simulink model "Test_model_671203"  (R2024a)
settings: Solver=VariableStepAuto  StartTime=0.0  StopTime=10  RelTol=1e-3
undefined symbols (not defined in the file or in its folder): X, Y, Z
libraries: sm_lib x63, nesl_utility x21
(part 3 of 3)

== matlab function Test_model_671203/MATLAB Function1 ==
  data: joint_angles input; x output; y output; z output
function [x, y, z] = FK_Simulink(joint_angles)
    % FK_Simulink: Calculates the position and orientation of the end effector for a 4-DOF manipulator

    % Lengths of the links
    d1 = 0.3;  % {0} -> {1}
    a1 = 0.2;  % {1} -> {2}
    L1 = 0.25; % Link 1
    L2 = 1;    % Link 2
    L3 = 1.5;  % Link 3
    L4 = 0.75; % Link 4 (End Effector)

    % Extract joint angles
    q1 = joint_angles(1); % Joint 1 (base rotation)
    q2 = joint_angles(2); % Joint 2 (shoulder rotation)
    q3 = joint_angles(3); % Joint 3 (elbow rotation)
    q4 = joint_angles(4); % Joint 4 (end effector orientation)

    x12 = pi/2;
    z23 = pi/2;

    % Transformation Matrices
    % Transform from base frame to end effector
    % Transformation for Joint 0 -> 1 (Rotation around the base)
    T01_T1 = [  1, 0, 0,  0;
                0, 1, 0,  0;
                0, 0, 1, d1;
                0, 0, 0,  1];

    T01_Rz = [  cos(q1), -sin(q1), 0, 0;
                sin(q1),  cos(q1), 0, 0;
                      0,        0, 1, 0;
                      0,        0, 0, 1];

    T01 = T01_T1 * T01_Rz;

    % Transformation for Joint 1 -> 2 (shoulder)
    T12_T1 = [  1, 0, 0, -a1;
                0, 1, 0,   0;
                0, 0, 1,  L1;
                0, 0, 0,   1];

    T12_Rx = [  1,        0,         0, 0;
                0, cos(x12), -sin(x12), 0;
                0, sin(x12),  cos(x12), 0;
                0,        0,         0, 1];

    T12_Rz = [  cos(q2), -sin(q2), 0, 0;
                sin(q2),  cos(q2), 0, 0;
                      0,        0, 1, 0;
                      0,        0, 0, 1];

    T12 = T12_T1 * T12_Rx * T12_Rz;

    % Transformation for Joint 2 -> 3 (elbow)
    T23_Rz1 = [  cos(z23), -sin(z23), 0, 0;
                 sin(z23),  cos(z23), 0, 0;
                        0,         0, 1, 0;
                        0,         0, 0, 1];

    T23_T1 = [  1, 0, 0, L2;
                0, 1, 0,  0;
                0, 0, 1,  0;
                0, 0, 0,  1];

    T23_Rz = [  cos(q3), -sin(q3), 0, 0;
                sin(q3),  cos(q3), 0, 0;
                      0,        0, 1, 0;
                      0,        0, 0, 1];

    T23 = T23_Rz1 * T23_T1 * T23_Rz;

    % Transformation for Joint 3 -> 4
    T34_T1 = [  1, 0, 0, L3;
                0, 1, 0,  0;
                0, 0, 1,  0;
                0, 0, 0,  1];

    T34_Rz = [  cos(q4), -sin(q4), 0, 0;
                sin(q4),  cos(q4), 0, 0;
                      0,        0, 1, 0;
                      0,        0, 0, 1];

    T34 = T34_T1 * T34_Rz;

    % Transformation for Joint 4 -> e

    T4e = [ 1, 0, 0, L4;
            0, 1, 0,  0;
            0, 0, 1,  0;
            0, 0, 0,  1];

    % Final transformation from the base to end effector
    T = T01 * T12 * T23 * T34 * T4e;

    % Extract position from the final transformation matrix
    x = T(1, 4); % x-position of the end effector
    y = T(2, 4); % y-position of the end effector
    z = T(3, 4); % z-position of the end effector

  
end

% Tranformation matrix
% ([  [-sin(q2 + q3 + q4)*cos(q1), -cos(q1)*cos(q2 + q3 + q4),  sin(q1), -L2*sin(q2)*cos(q1) - L3*sin(q2 + q3)*cos(q1) - L4*sin(q2 + q3 + q4)*cos(q1) - a1*cos(q1)], ...
%     [-sin(q1)*sin(q2 + q3 + q4), -sin(q1)*cos(q2 + q3 + q4), -cos(q1), -L2*sin(q1)*sin(q2) - L3*sin(q1)*sin(q2 + q3) - L4*sin(q1)*sin(q2 + q3 + q4) - a1*sin(q1)], ...
%     [         cos(q2 + q3 + q4),         -sin(q2 + q3 + q4),        0,                     L1 + L2*cos(q2) + L3*(1.0*cos(q2 + q3)) + L4*(cos(q2 + q3 + q4)) + d1], ...
%     [                         0,                          0,        0,                                                                                         1]  ])


function q = solveMatrix(x, y, z, phi)
    % Define matrices A, B, C, D, E (as 4x4 symbolic matrices)
    syms x y z phi real;
    
     % Lengths of the links
    d1 = 0.3;  % {0} -> {1}
    a1 = 0.2;  % {1} -> {2}
    L1 = 0.25; % Link 1
    L2 = 1;    % Link 2
    L3 = 1.5;  % Link 3
    L4 = 0.75; % Link 4 (End Effector)

    % Extract joint angles
    q1 = joint_angles(1); % Joint 1 (base rotation)
    q2 = joint_angles(2); % Joint 2 (shoulder rotation)
    q3 = joint_angles(3); % Joint 3 (elbow rotation)
    q4 = joint_angles(4); % Joint 4 (end effector orientation)

    x12 = pi/2;
    z23 = pi/2;

    % Transformation Matrices
    % Transform from base frame to end effector
    % Transformation for Joint 0 -> 1 (Rotation around the base)
    T01_T1 = [  1, 0, 0,  0;
                0, 1, 0,  0;
                0, 0, 1, d1;
                0, 0, 0,  1];

    T01_Rz = [  cos(q1), -sin(q1), 0, 0;
                sin(q1),  cos(q1), 0, 0;
                      0,        0, 1, 0;
                      0,        0, 0, 1];

    T01 = T01_T1 * T01_Rz;

    % Transformation for Joint 1 -> 2 (shoulder)
    T12_T1 = [  1, 0, 0, -a1;
                0, 1, 0,   0;
                0, 0, 1,  L1;
                0, 0, 0,   1];

    T12_Rx = [  1,        0,         0, 0;
                0, cos(x12), -sin(x12), 0;
                0, sin(x12),  cos(x12), 0;
                0,        0,         0, 1];

    T12_Rz = [  cos(q2), -sin(q2), 0, 0;
                sin(q2),  cos(q2), 0, 0;
                      0,        0, 1, 0;
                      0,        0, 0, 1];

    T12 = T12_T1 * T12_Rx * T12_Rz;

    % Transformation for Joint 2 -> 3 (elbow)
    T23_Rz1 = [  cos(z23), -sin(z23), 0, 0;
                 sin(z23),  cos(z23), 0, 0;
                        0,         0, 1, 0;
                        0,         0, 0, 1];

    T23_T1 = [  1, 0, 0, L2;
                0, 1, 0,  0;
                0, 0, 1,  0;
                0, 0, 0,  1];

    T23_Rz = [  cos(q3), -sin(q3), 0, 0;
                sin(q3),  cos(q3), 0, 0;
                      0,        0, 1, 0;
                      0,        0, 0, 1];

    T23 = T23_Rz1 * T23_T1 * T23_Rz;

    % Transformation for Joint 3 -> 4
    T34_T1 = [  1, 0, 0, L3;
                0, 1, 0,  0;
                0, 0, 1,  0;
                0, 0, 0,  1];

    T34_Rz = [  cos(q4), -sin(q4), 0, 0;
                sin(q4),  cos(q4), 0, 0;
                      0,        0, 1, 0;
                      0,        0, 0, 1];

    T34 = T34_T1 * T34_Rz;

    % Transformation for Joint 4 -> e

    T4e = [ 1, 0, 0, L4;
            0, 1, 0,  0;
            0, 0, 1,  0;
            0, 0, 0,  1];

    % Final transformation from the base to end effector
    T = T01 * T12 * T23 * T34 * T4e;
    
    % Define result matrix X (4x4)
    X = [-sin(q2 + q3 + q4)*cos(q1), -cos(q1)*cos(q2 + q3 + q4),  sin(q1), -L2*sin(q2)*cos(q1) - L3*sin(q2 + q3)*cos(q1) - L4*sin(q2 + q3 + q4)*cos(q1) - a1*cos(q1); ...
         -sin(q1)*sin(q2 + q3 + q4), -sin(q1)*cos(q2 + q3 + q4), -cos(q1), -L2*sin(q1)*sin(q2) - L3*sin(q1)*sin(q2 + q3) - L4*sin(q1)*sin(q2 + q3 + q4) - a1*sin(q1); ...
                  cos(q2 + q3 + q4),         -sin(q2 + q3 + q4),        0,                     L1 + L2*cos(q2) + L3*(1.0*cos(q2 + q3)) + L4*(cos(q2 + q3 + q4)) + d1; ...
                                  0,                          0,        0,                                                                                         1];
    
    % Solve the equation A*B*C*D*E = X
    eqn = T == X;
    q = solve(eqn, [q1, q2, q3, q4]);
end

== matlab function Test_model_671203/MATLAB Function5 ==
  data: x input; solutions output; y input; z input
%#codegen
function solutions = solveMatrix(x, y, z)
    % กำหนดขนาดคงที่สำหรับ output solutions
    solutions = zeros(1, 4); % solutions จะมีขนาด [1x4] เสมอ

    % Lengths of the links
    d1 = 0.3;  
    a1 = 0.2;  
    L1 = 0.25; 
    L2 = 1;    
    L3 = 1.5;  
    L4 = 0.75; 

    % Initial guess for q1, q2, q3, q4
    initial_guess = [0, 0, 0, 0];

    % Define the function to solve
    function F = equations(vars)
        q1 = vars(1);
        q2 = vars(2);
        q3 = vars(3);
        q4 = vars(4);
        F = [
            -L2*sin(q2)*cos(q1) - L3*sin(q2 + q3)*cos(q1) - L4*sin(q2 + q3 + q4)*cos(q1) - a1*cos(q1) - x;
            -L2*sin(q1)*sin(q2) - L3*sin(q1)*sin(q2 + q3) - L4*sin(q1)*sin(q2 + q3 + q4) - a1*sin(q1) - y;
            L1 + L2*cos(q2) + L3*cos(q2 + q3) + L4*cos(q2 + q3 + q4) + d1 - z;
        ];
    end

    % Solve the equations numerically
    options = optimoptions('fsolve', 'Algorithm', 'levenberg-marquardt', 'Display', 'none');
    solutions = fsolve(@equations, initial_guess, options);
end
